simulink model "exhaust_fan_speed_logic"  (R2020b)
settings: Solver=VariableStepAuto  StartTime=0.0  StopTime=inf  RelTol=1e-3
settings Model: DataDictionary=airsys_data_dict.sldd  Creator=Litao  LastModifiedBy=Litao

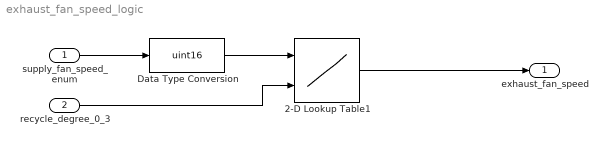
== system exhaust_fan_speed_logic ==
  supply_fan_speed_enum : Inport  OutDataTypeStr=Enum: fan_speed_enum
  recycle_degree_0_3 : Inport  Port=2  OutDataTypeStr=uint16
  2-D Lookup Table1 : Lookup_n-D  BreakpointsForDimension1=uint16([1,2,3]);  BreakpointsForDimension2=uint16([0,1,2,3]);  Table=uint16(reshape([100,200,300,110,210,310,120,220,320,130,230,330],3,4));  ExtrapMethod=Clip  InternalRulePriority=Speed  RndMeth=Simplest  InputSameDT=on
      settings: InputPortMap=u0,u1
  Data Type Conversion : DataTypeConversion  OutDataTypeStr=uint16
  exhaust_fan_speed : Outport
  wires:
  supply_fan_speed_enum/1 -> Data Type Conversion/1
  recycle_degree_0_3/1 -> 2-D Lookup Table1/2
  Data Type Conversion/1 -> 2-D Lookup Table1/1
  2-D Lookup Table1/1 -> exhaust_fan_speed/1
